simulink model "neckLinAngVel"  (Simulink 8.3)
settings: Solver=FixedStepDiscrete  StartTime=0.0  StopTime=inf  FixedStep=Ts  RelTol=1e-3
undefined symbols (not defined in the file): localName, robotName, Ts
libraries: WBCLibrary x11
settings Model: Creator=jorhabib  LastModifiedBy=jorhabib
settings DataIOCC: SignalLoggingSaveFormat=Dataset
settings DebuggingCC: UnderspecifiedInitializationDetection=Simplified  StateNameClashWarn=none
settings GRTTargetCC: CombineOutputUpdateFcns=on  GRTInterface=off

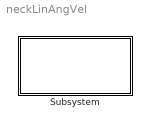
== system neckLinAngVel ==
  Subsystem : Subsystem  mask{robotName=robotName, localName=localName, Ts=Ts}
      mask prompts: robotName "Robot name"; localName "Local name"

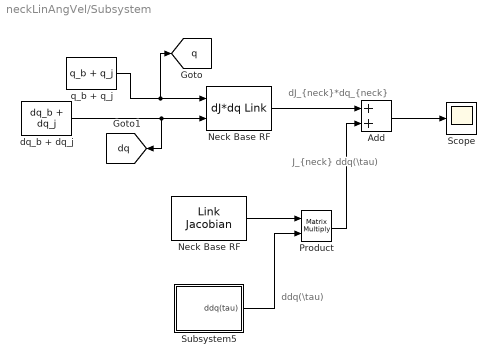
== system neckLinAngVel/Subsystem ==
  note: ddq(\tau)
  note: J_{neck} ddq(\tau)
  note: dJ_{neck}*dq_{neck}
  Add : Sum
  Neck Base RF : WBCLibrary/wholeBodyModel/Dynamics/dJ*dq Link  val=19  robotName=robotName  localName=localName  link=chest
  "Neck Base RF " : WBCLibrary/wholeBodyModel/Jacobians/Link Jacobian  robotname=robotName  localname=localName  link=chest
  Product : Product  Multiplication=Matrix(*)
  Scope : Scope
      settings: ShowLegends=on
  Subsystem5 : Subsystem
  dq_b + dq_j : WBCLibrary/wholeBodyStates/dq_b + dq_j
  q_b + q_j : WBCLibrary/wholeBodyStates/q_b + q_j
  tag scope: dq=global, q=global
  wires:
  Product/1 -> Add/2
  Neck Base RF/1 -> Add/1
  Add/1 -> Scope/1
  dq_b + dq_j/1 -> [dq], Neck Base RF/2
  q_b + q_j/1 -> [q], Neck Base RF/1
  Subsystem5/1(ddq(tau)) -> Product/2
  "Neck Base RF "/1 -> Product/1

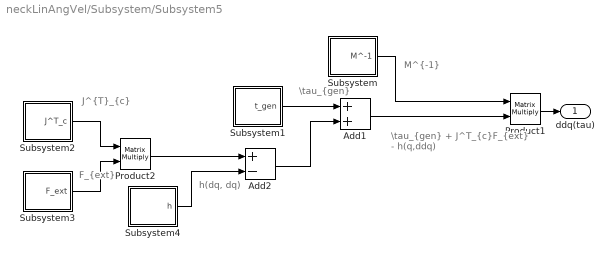
== system neckLinAngVel/Subsystem/Subsystem5 ==
  note: \tau_{gen} + J^T_{c}F_{ext} - h(q,ddq)
  note: h(dq, dq)
  note: J^{T}_{c}
  note: M^{-1}
  note: F_{ext}
  note: \tau_{gen}
  Add1 : Sum  SampleTime=Ts
  Add2 : Sum  Inputs=+-  SampleTime=Ts
  Product1 : Product  Multiplication=Matrix(*)  SampleTime=Ts
  Product2 : Product  Multiplication=Matrix(*)  SampleTime=Ts
  Subsystem : Subsystem
  Subsystem1 : Subsystem
  Subsystem2 : Subsystem
  Subsystem3 : Subsystem
  Subsystem4 : Subsystem
  ddq(tau) : Outport
  wires:
  Subsystem2/1(J^T_c) -> Product2/1
  Subsystem3/1(F_ext) -> Product2/2
  Product2/1 -> Add2/1
  Subsystem1/1(t_gen) -> Add1/1
  Product1/1 -> ddq(tau)/1
  Add2/1 -> Add1/2
  Subsystem/1(M^-1) -> Product1/1
  Subsystem4/1(h) -> Add2/2
  Add1/1 -> Product1/2

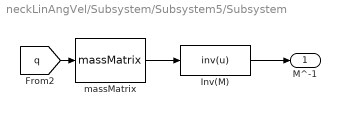
== system neckLinAngVel/Subsystem/Subsystem5/Subsystem ==
  Inv(M) : MATLABFcn  MATLABFcn=inv(u)  Output1D=off  SampleTime=Ts
  massMatrix : WBCLibrary/wholeBodyModel/Dynamics/massMatrix  val=8  robotname=robotName  localname=localName
  M^-1 : Outport
  wires:
  [q] -> massMatrix/1
  Inv(M)/1 -> M^-1/1
  massMatrix/1 -> Inv(M)/1

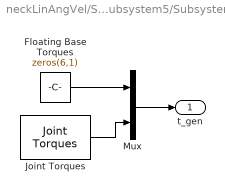
== system neckLinAngVel/Subsystem/Subsystem5/Subsystem1 ==
  Floating Base Torques : Constant  Value=zeros(6,1)  SampleTime=Ts
  Joint Torques : WBCLibrary/wholeBodyStates/Joint Torques  robotName=robotName  localName=localName
  Mux : Mux  Inputs=2
  t_gen : Outport
  wires:
  Joint Torques/1 -> Mux/2
  Floating Base Torques/1 -> Mux/1
  Mux/1 -> t_gen/1

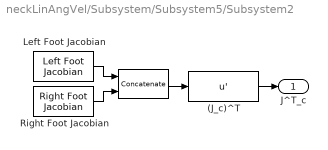
== system neckLinAngVel/Subsystem/Subsystem5/Subsystem2 ==
  " " : Concatenate  Mode=Multidimensional array
  (J_c)^T : MATLABFcn  MATLABFcn=u'  Output1D=off  SampleTime=Ts
  Left Foot Jacobian : WBCLibrary/wholeBodyModel/Jacobians/Left Foot Jacobian  robotName=robotName  localName=localName
  Right Foot Jacobian : WBCLibrary/wholeBodyModel/Jacobians/Right Foot Jacobian  robotName=robotName  localName=localName
  J^T_c : Outport
  wires:
  (J_c)^T/1 -> J^T_c/1
  " "/1 -> (J_c)^T/1
  Right Foot Jacobian/1 -> " "/2
  Left Foot Jacobian/1 -> " "/1

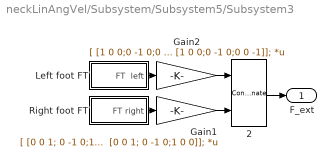
== system neckLinAngVel/Subsystem/Subsystem5/Subsystem3 ==
  " 2" : Concatenate  Mode=Multidimensional array
  Gain1 : Gain  Gain="[ [0 0 1; 0 -1 0;1 0 0], zeros(3,3); zeros(3,3),  [0 0 1; 0 -1 0;1 0 0]];"  Multiplication=Matrix(K*u)  SampleTime=Ts
  Gain2 : Gain  Gain="[ [1 0 0;0 -1 0;0 0 -1], zeros(3,3); zeros(3,3),  [1 0 0;0 -1 0;0 0 -1]];"  Multiplication=Matrix(K*u)  SampleTime=Ts
  Left foot FT : Subsystem
  Right foot FT : Subsystem
  F_ext : Outport
  wires:
  Right foot FT/1(FT right) -> Gain1/1
  Left foot FT/1(FT  left) -> Gain2/1
  Gain2/1 -> " 2"/1
  Gain1/1 -> " 2"/2
  " 2"/1 -> F_ext/1

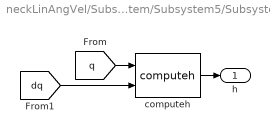
== system neckLinAngVel/Subsystem/Subsystem5/Subsystem4 ==
  computeh : WBCLibrary/wholeBodyModel/Dynamics/computeh  val=7  robotname=robotName  localname=localName
  h : Outport
  wires:
  [q] -> computeh/1
  computeh/1 -> h/1
  [dq] -> computeh/2

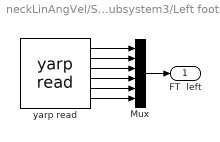
== system neckLinAngVel/Subsystem/Subsystem5/Subsystem3/Left foot FT ==
  Mux : Mux  Inputs=6
  yarp read : WBCLibrary/Utilities/yarp read  from='/icub/left_foot/analog:o'  to='...'  num=6
  FT  left : Outport
  wires:
  yarp read/1 -> Mux/1
  yarp read/2 -> Mux/2
  yarp read/3 -> Mux/3
  yarp read/4 -> Mux/4
  yarp read/5 -> Mux/5
  yarp read/6 -> Mux/6
  Mux/1 -> FT  left/1

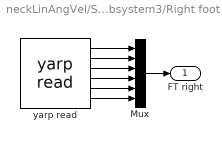
== system neckLinAngVel/Subsystem/Subsystem5/Subsystem3/Right foot FT ==
  Mux : Mux  Inputs=6
  yarp read : WBCLibrary/Utilities/yarp read  from='/icub/right_foot/analog:o'  to='...'  num=6
  FT right : Outport
  wires:
  yarp read/1 -> Mux/1
  yarp read/2 -> Mux/2
  yarp read/3 -> Mux/3
  yarp read/4 -> Mux/4
  yarp read/5 -> Mux/5
  yarp read/6 -> Mux/6
  Mux/1 -> FT right/1
